simulink model "PID_diagram"  (Simulink 7.7)
settings: Solver=ode45  StartTime=0.0  StopTime=10.0  RelTol=1e-3
values from neighbouring files (symbols this model uses):
  D = triu(qr(D))    [MgnCalibration.m]
  I = eye(length(P))    [EKF.m]    (also in EKF2.m; EKF2Simple.m; EKFSimple.m; kalman4.m = [1 0 0 0)
  P = (I - K*H)*P    [EKF.m]    (also in EKF2.m; EKF2Simple.m; EKFSimple.m; kalman4.m)
settings Model: Creator=Matt  LastModifiedBy=Matt
settings RTWCC: TargetLang=C++

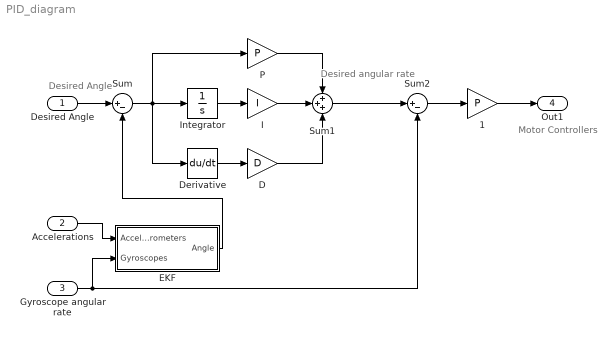
== system PID_diagram ==
  note: Motor Controllers
  note: Desired
      | angular rate
  note: Desired Angle
  Desired Angle : Inport
  Accelerations : Inport  Port=2
  Gyroscope angular rate : Inport  Port=3
  1 : Gain  Gain=P
  D : Gain  Gain=D
  Derivative : Derivative
  EKF : Subsystem
  I : Gain  Gain=I
  Integrator : Integrator
  P : Gain  Gain=P
  Sum : Sum  Inputs=|+-
  Sum1 : Sum  Inputs=+++
  Sum2 : Sum  Inputs=|+-
  Out1 : Outport  Port=4
  wires:
  Sum/1 -> Integrator/1, P/1, Derivative/1
  Derivative/1 -> D/1
  Integrator/1 -> I/1
  P/1 -> Sum1/1
  I/1 -> Sum1/2
  D/1 -> Sum1/3
  Sum1/1 -> Sum2/1
  Sum2/1 -> 1/1
  1/1 -> Out1/1
  Desired Angle/1 -> Sum/1
  EKF/1(Angle) -> Sum/2
  Accelerations/1 -> EKF/1(Accelerometers)
  Gyroscope angular rate/1 -> Sum2/2, EKF/2(Gyroscopes)

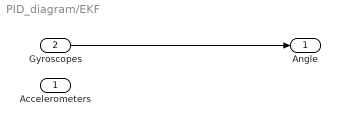
== system PID_diagram/EKF ==
  Accelerometers : Inport
  Gyroscopes : Inport  Port=2
  Angle : Outport
  wires:
  Gyroscopes/1 -> Angle/1
